simulink model "blockdemo"  (Simulink 6.3)
settings: Solver=VariableStepDiscrete  StartTime=0  StopTime=25  FixedStep=1  RelTol=1e-3
InitFcn:
  | %% DSPBuilder Start
  | alt_dspbuilder_update_model(bdroot)
  | %% DSPBuilder End
libraries: allblocks_alteradspbuilder2 x9, simulink x1
settings Model: Creator=mjervis  LastModifiedBy=delphick
settings DebuggingCC: MultiTaskDSMMsg=error

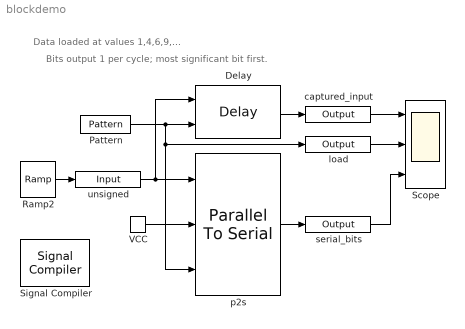
== system blockdemo ==
  note: Data loaded at values 1,4,6,9,...
  note: Bits output 1 per cycle; most significant bit first.
  Delay : allblocks_alteradspbuilder2/Delay  pipeline=1  ClockPhase=1  use_ena=on  use_sclr=off
  Pattern : allblocks_alteradspbuilder2/Pattern  Sequence=10000  SpecifyClock=off  use_ena=off  use_sclr=off
  Ramp2 : simulink/Sources/Ramp  slope=0.5  start=0  X0=1
      settings: AttributesFormatString=slope = %<slope>\nx0 = %<X0>
  Scope : Scope  NumInputPorts=3
      settings: YMin=-1~-0.5~-0.5  YMax=10~1.5~1.5  SaveName=ScopeData4
  Signal Compiler : allblocks_alteradspbuilder2/Signal Compiler  DeviceFamily=Stratix IV  DeviceName=AUTO  EnableSignalTap=off  SignalTapDepth=128  UseBoardBlock=off  StpUseDefaultClock=on  StpClock=clock
  VCC : allblocks_alteradspbuilder2/VCC  SpecifyClock=off
  captured_input : allblocks_alteradspbuilder2/Output  iofile=C:\workspace_clean\Documentation\DesignExamples\Tutorials\UnitBlocks\Storage\ParallelToSerial\tb_blockdemo\blockdemo_captured_input.capture  BusType=Unsigned Integer  bwl=4  bwr=0  PORTTYPE=Output
  load : allblocks_alteradspbuilder2/Output  iofile=C:\workspace_clean\Documentation\DesignExamples\Tutorials\UnitBlocks\Storage\ParallelToSerial\tb_blockdemo\blockdemo_load.capture  BusType=Unsigned Integer  bwl=4  bwr=0  PORTTYPE=Output
  p2s : allblocks_alteradspbuilder2/Parallel To Serial  BusType=Unsigned Integer  bwl=4  bwr=0  msbfirsttext=MSB First  msbfirst=1  repeatlastbit=off  use_sclr=off
  serial_bits : allblocks_alteradspbuilder2/Output  iofile=C:\workspace_clean\Documentation\DesignExamples\Tutorials\UnitBlocks\Storage\ParallelToSerial\tb_blockdemo\blockdemo_serial_bits.capture  BusType=Single Bit  bwl=8  bwr=0  PORTTYPE=Output
  unsigned : allblocks_alteradspbuilder2/Input  iofile=C:\workspace_clean\Documentation\DesignExamples\Tutorials\UnitBlocks\Storage\ParallelToSerial\tb_blockdemo\blockdemo_unsigned.salt  BusType=Unsigned Integer  bwl=4  bwr=0  SpecifyClock=off  clock=default_clock  PORTTYPE=Input
  wires:
  Pattern/1 -> Delay/2, p2s/3, load/1
  VCC/1 -> p2s/2
  Ramp2/1 -> unsigned/1
  unsigned/1 -> p2s/1, Delay/1
  serial_bits/1 -> Scope/3
  p2s/1 -> serial_bits/1
  Delay/1 -> captured_input/1
  captured_input/1 -> Scope/1
  load/1 -> Scope/2
